simulink model "s6_HESG"  (R2019b)
settings: Solver=VariableStepAuto  StartTime=0.0  StopTime=15  RelTol=1e-3
libraries: powerlib x4, powerlib_meascontrol x2, fuzblock x1, simulink_extras x1
settings Model: SimulationMode=accelerator  Creator=MAHMUD  LastModifiedBy=MAHMUD
settings SolverCC: ZeroCrossAlgorithm=Adaptive
settings DebuggingCC: IgnoredZcDiagnostic=none

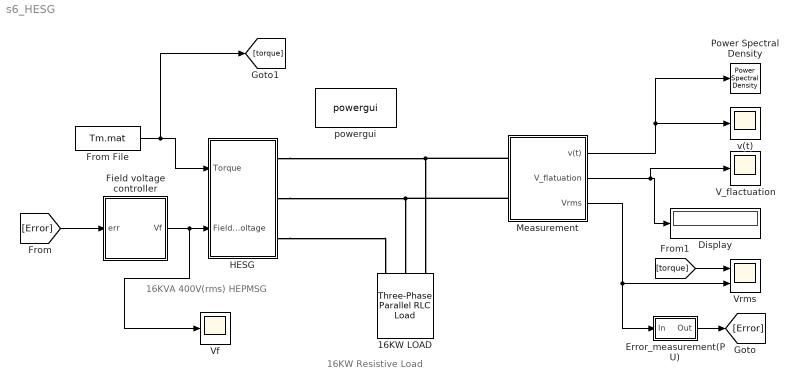
== system s6_HESG ==
  note: 16KVA 400V(rms) HEPMSG
  note: 16KW Resistive Load
  16KW LOAD : powerlib/Elements/Three-Phase Parallel RLC Load  LConnTagsString=A|B|C  Configuration=Y (grounded)  NominalVoltage=400  Vabc=[1e3 1e3 1e3]  Vabcp=[1e3 1e3 1e3]  NominalFrequency=50  UnbalancedPower=off  ActivePower=16e3  InductivePower=0  CapacitivePower=0  Pabc=[10e3 9e3 11e3]  QLabc=[100 90 110]  QCabc=[100 90 110]  Pabcp=[10e3 9e3 11e3]  QLabcp=[100 90 110]  QCabcp=[100 90 110]  Measurements=None  LoadType=constant PQ
      settings: SourceProductName=Simscape Electrical
  Display : Display
  Error_measurement(PU) : Subsystem
  Field voltage controller : Subsystem
  From File : FromFile  FileName=Tm.mat  SampleTime=0
  HESG : Subsystem
  Measurement : Subsystem
  Power Spectral Density : simulink_extras/Additional Sinks/Power Spectral Density  npts=5000  fftpts=512  HowOften=500  sampleT=0.001
      settings: SourceProductName=Simulink  SourceProductBaseCode=SL
  V_flactuation : Scope
  Vf : Scope
  Vrms : Scope  NumInputPorts=2
  powergui : powerlib/powergui  Priority=1  SimulationMode=Continuous  SampleTime=50e-6  frequency=60  Iterations=50  frequencyindice=50  Pbase=100e6  ErrMax=1e-4  UnitsV=kV  UnitsW=MW  buscounter=0  FunctionMessages=off  echomessages=off  EnableUseOfTLC=off  CurrentSourceSwitches=off  DisableSnubberDevices=off  DisableRonSwitches=off  DisableVfSwitches=off  DisplayEquations=off  AutomaticDiscreteSolvers=off  SolverType=Tustin/Backward Euler (TBE)  Interpol=off  ExternalGateDelay=off  methode=off  Ts=100  x0status=blocks  SPID=on  SwTol=0  HookPort=off  NonlinearTolerance=1e-4  nMaxIteration=100  ContinueOnMaxIteration=off  RestoreLinks=warning  ResistiveCurrentMeasurement=off  Frange=[0:2:500]  Ylog=off  Xlog=on  ShowGrid=off  save=off  variable=ZData  structure=0  ZoomFFT=off  StartTime=0.0  cycles=1  DisplayStyle=1  fundamental=60  FreqAxis=off  MaxFrequency=1000  frequencyindicesteady=1  RmsSteady=1  display=off
      settings: SourceProductName=Simscape Electrical
  v(t) : Scope
  wires:
  From File/1 -> [torque], HESG/1(Torque)
  [Error] -> Field voltage controller/1(err)
  Field voltage controller/1(Vf) -> Vf/1, HESG/2(Field voltage)
  Error_measurement(PU)/1(Out) -> [Error]
  Measurement/1(v(t)) -> v(t)/1, Power Spectral Density/1
  Measurement/2(V_flatuation) -> Display/1, V_flactuation/1
  Measurement/3(Vrms) -> Vrms/2, Error_measurement(PU)/1(In)
  [torque] -> Vrms/1
  connections:
  HESG/RConn3 -- 16KW LOAD/LConn1
  HESG/RConn1 -- Measurement/LConn1 -- 16KW LOAD/LConn3
  HESG/RConn2 -- 16KW LOAD/LConn2 -- Measurement/LConn2

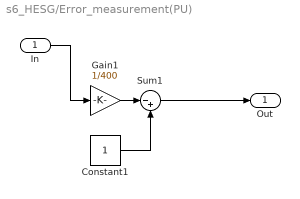
== system s6_HESG/Error_measurement(PU) ==
  In : Inport
  Constant1 : Constant
  Gain1 : Gain  Gain=1/400
  Sum1 : Sum  Inputs=|-+
  Out : Outport
  wires:
  In/1 -> Gain1/1
  Gain1/1 -> Sum1/1
  Constant1/1 -> Sum1/2
  Sum1/1 -> Out/1

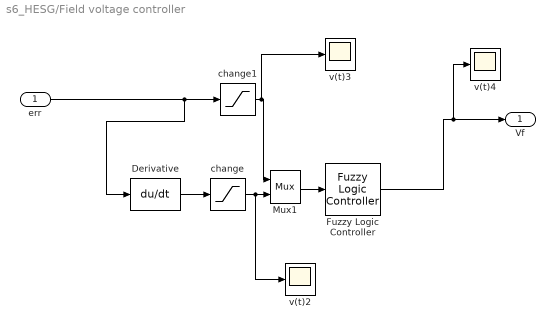
== system s6_HESG/Field voltage controller ==
  err : Inport
  Derivative : Derivative
  Fuzzy Logic Controller : fuzblock/Fuzzy Logic  Controller  FIS='VC.fis'  OutputSampleNumber=101  DataType=double  FuzzifiedInputs=off  RuleFiringStrengths=off  RuleOutputs=off  AggregatedOutputs=off  SimulateUsing=Interpreted execution  OutOfRangeInputValueMessage=warning  NoRuleFiredMessage=warning  EmptyOutputFuzzySetMessage=warning
  Mux1 : Mux  Inputs=2
  change : Saturate  UpperLimit=1  LowerLimit=-1  ZeroCross=off
  change1 : Saturate  UpperLimit=0.1  LowerLimit=-0.05  ZeroCross=off
  v(t)2 : Scope
  v(t)3 : Scope
  v(t)4 : Scope
  Vf : Outport
  wires:
  change/1 -> v(t)2/1, Mux1/2
  Derivative/1 -> change/1
  change1/1 -> v(t)3/1, Mux1/1
  Fuzzy Logic Controller/1 -> v(t)4/1, Vf/1
  err/1 -> change1/1, Derivative/1
  Mux1/1 -> Fuzzy Logic Controller/1

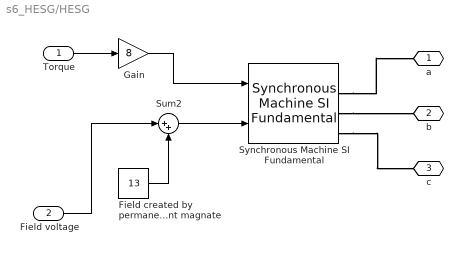
== system s6_HESG/HESG ==
  Torque : Inport
  Field voltage : Inport  Port=2
  "Field created by permanent magnate " : Constant  Value=13
  Gain : Gain  Gain=8
  Sum2 : Sum  Inputs=|++
  Synchronous Machine SI Fundamental : powerlib/Machines/Synchronous Machine SI Fundamental  PresetModel=No  MechanicalLoad=Mechanical power Pm  ShowDetailedParameters=on  RotorType=Salient-pole  Units=SI fundamental parameters  MeasurementBus=off  NominalParameters=[1.6e+04 400 50]  Stator=[0.645 0.002228 0.05297 0.02518]  Field=[0.3968 0.005492]  Dampers2=[ 0.0664, 1.387e-3, 0.0292, 6.896e-4, 7.907e-3, 2.477e-3]  Dampers1=[0.9843 0.003371 1.545 0.004906]  Mechanical=[0.1278 0.013 1]  PolePairs=2  InitialConditions="[ 0  0  0  0  0  0  0  0  70.3192 ]"  SetSaturation=off  Saturation=[695.64,774.7,917.5,1001.6,1082.2,1175.9,1293.6,1430.2,1583.7;9660,10623,12243,13063,13757,14437,15180,15890,16567]  DisplayVfd=off  LoadFlowParameters=[1,0,0,0,0]  TsPowergui=0  TsBlock=-1  IterativeModel=Trapezoidal non iterative  IterativeDiscreteModel=Trapezoidal non iterative  BusType=PV  Pref=0  Qref=0  Qmin=-inf  Qmax=inf  PLF=0  QLF=0
      settings: SourceProductName=Simscape Electrical  SourceProductBaseCode=PS
  a : PMIOPort  Side=Right
  b : PMIOPort  Port=2  Side=Right
  c : PMIOPort  Port=3  Side=Right
  wires:
  Gain/1 -> Synchronous Machine SI Fundamental/1
  Sum2/1 -> Synchronous Machine SI Fundamental/2
  "Field created by permanent magnate "/1 -> Sum2/2
  Field voltage/1 -> Sum2/1
  Torque/1 -> Gain/1
  connections:
  Synchronous Machine SI Fundamental/RConn2 -- b/RConn1
  Synchronous Machine SI Fundamental/RConn3 -- c/RConn1
  Synchronous Machine SI Fundamental/RConn1 -- a/RConn1

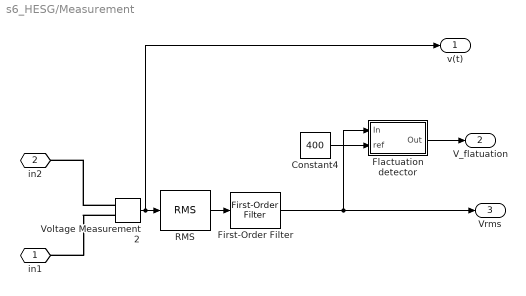
== system s6_HESG/Measurement ==
  Constant4 : Constant  Value=400
  First-Order Filter : powerlib_meascontrol/Filters/First-Order Filter  FilterType=Lowpass  Tc=100e-3  Ts=0  Initialize=off  Vac_Init=[0, 0, 50]  Vdc_Init=0  PlotResponse=off  FreqRange="[0,  200,  1]"
      settings: SourceProductName=Simscape Electrical
  Flactuation detector : Subsystem
  RMS : powerlib_meascontrol/Measurements/RMS  TrueRMS=on  Freq=50  RMSInit=210  Ts=0.001
      settings: SourceProductName=Simscape Electrical
  Voltage Measurement2 : powerlib/Measurements/Voltage Measurement  PhasorSimulation=off  OutputType=Complex  PSBequivalent=0
      settings: SourceProductName=Simscape Electrical
  in1 : PMIOPort  Side=Left
  in2 : PMIOPort  Port=2  Side=Left
  v(t) : Outport
  V_flatuation : Outport  Port=2
  Vrms : Outport  Port=3
  wires:
  Voltage Measurement2/1 -> v(t)/1, RMS/1
  First-Order Filter/1 -> Flactuation detector/1(In), Vrms/1
  RMS/1 -> First-Order Filter/1
  Flactuation detector/1(Out) -> V_flatuation/1
  Constant4/1 -> Flactuation detector/2(ref)
  connections:
  Voltage Measurement2/LConn2 -- in1/RConn1
  Voltage Measurement2/LConn1 -- in2/RConn1

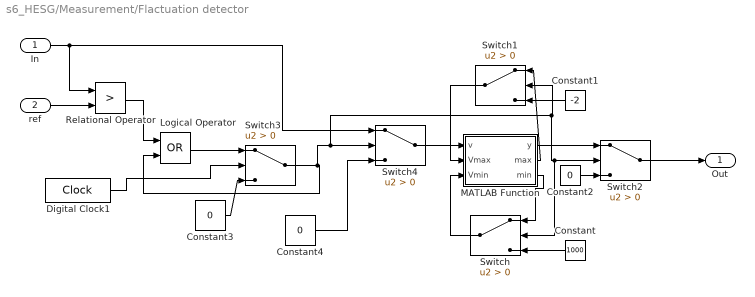
== system s6_HESG/Measurement/Flactuation detector ==
  In : Inport
  ref : Inport  Port=2
  Constant : Constant  Value=1000
  Constant1 : Constant  Value=-2
  Constant2 : Constant  Value=0
  Constant3 : Constant  Value=0
  Constant4 : Constant  Value=0
  Digital Clock1 : DigitalClock
  Logical Operator : Logic  Operator=OR  AllPortsSameDT=off  OutDataTypeStr=boolean
  MATLAB Function : MATLAB Function  TreatAsAtomicUnit=on
  Relational Operator : RelationalOperator  Operator=>  OutDataTypeStr=boolean  ZeroCross=off  RndMeth=Simplest
  Switch{,1..4} (5 alike) : Switch  Criteria=u2 > Threshold  ZeroCross=off
  Out : Outport
  wires:
  Constant/1 -> Switch/3
  Switch1/1 -> MATLAB Function/2(Vmax)
  Constant1/1 -> Switch1/3
  MATLAB Function/1(y) -> Switch2/1
  MATLAB Function/3(min) -> Switch/1
  Switch2/1 -> Out/1
  MATLAB Function/2(max) -> Switch1/1
  Switch/1 -> MATLAB Function/3(Vmin)
  Constant2/1 -> Switch2/3
  Logical Operator/1 -> Switch3/1
  Switch3/1 -> Switch/2, Switch2/2, Switch1/2, Switch4/2, Logical Operator/2
  Constant3/1 -> Switch3/3
  Relational Operator/1 -> Logical Operator/1
  Switch4/1 -> MATLAB Function/1(v)
  In/1 -> Relational Operator/1, Switch4/1
  Digital Clock1/1 -> Switch3/2
  ref/1 -> Relational Operator/2
  Constant4/1 -> Switch4/3

== matlab function s6_HESG/Measurement/Flactuation detector/MATLAB Function ==
  data: v input; y output; Vmax input; Vmin input; max output; min output
function [y,max,min] = fcn(v,Vmax,Vmin)
if(v>0)
    if(v<Vmin)
        min=v;
    else
        min=Vmin;
    end
    if(v>Vmax)
        max=v;
    else 
        max=Vmax;
    end
    y=Vmax-Vmin;
else
    min=0;
    max=0;
    y=0;
end
